simulink model "real_motor_model"  (R2023b)
settings: Solver=FixedStepAuto  StartTime=0.0  StopTime=2  FixedStep=0.0005  RelTol=1e-3
values from neighbouring files (symbols this model uses):
  dm = 0.0068    [params.m]
  Jm = 0.0104    [params.m]
settings Model: Creator=matte  LastModifiedBy=86180
settings SolverCC: AlgebraicLoopSolver=TrustRegion
settings DebuggingCC: ArithmeticOperatorsInVariantConditions=warning
settings SFSimCC: LegacyBehaviorForPersistentVarInContinuousTime=on  CustomCodeUndefinedFunction=UseInterfaceOnly

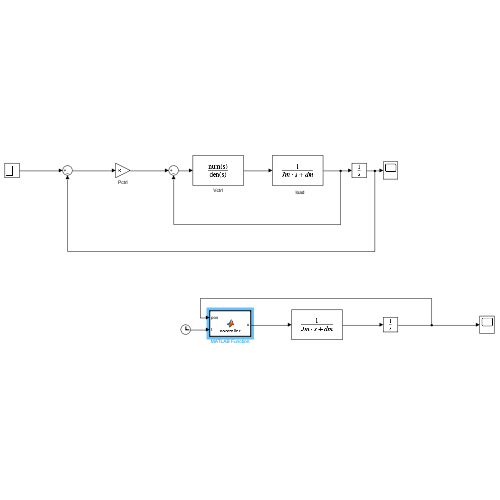
[thumbnail: Simulink's stored preview of the top-level diagram]
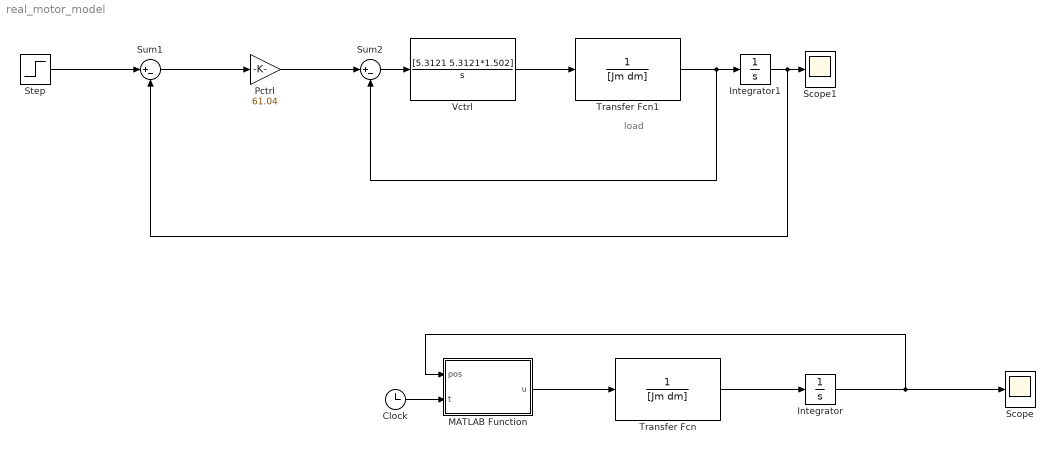
== system real_motor_model ==
  note: load
  Clock : Clock
  Integrator : Integrator
  Integrator1 : Integrator
  MATLAB Function : MATLAB Function  TreatAsAtomicUnit=on
  Pctrl : Gain  Gain=61.04
  Scope : Scope
  Scope1 : Scope
  Step : Step  SampleTime=0
  Sum1 : Sum  Inputs=|+-
  Sum2 : Sum  Inputs=|+-
  Transfer Fcn : TransferFcn  Denominator=[Jm dm]
  Transfer Fcn1 : TransferFcn  Denominator=[Jm dm]
  Vctrl : TransferFcn  Numerator=[5.3121 5.3121*1.502]  Denominator=[1 0]
  wires:
  Integrator/1 -> MATLAB Function/1(pos), Scope/1
  Transfer Fcn/1 -> Integrator/1
  Clock/1 -> MATLAB Function/2(t)
  MATLAB Function/1(u) -> Transfer Fcn/1
  Transfer Fcn1/1 -> Sum2/2, Integrator1/1
  Step/1 -> Sum1/1
  Vctrl/1 -> Transfer Fcn1/1
  Sum2/1 -> Vctrl/1
  Integrator1/1 -> Sum1/2, Scope1/1
  Pctrl/1 -> Sum2/1
  Sum1/1 -> Pctrl/1

== matlab function real_motor_model/MATLAB Function ==
  data: pos input; u output; t input
function u = controller(pos, t)

persistent last_t;
persistent last_pos;
persistent i_vel_e;

if isempty(last_pos)
    last_pos =pos;
end

% One time variable initialization --------
if isempty(last_t)
    last_t = 0;
end
% ----------------------------------------

if isempty(i_vel_e)
    i_vel_e = 0;
end

dt = t - last_t;

% Dirty fix to avoid division by zero --------
if dt == 0
    dt = 1e-4;
end

% --------------------------------------------
% implement your controller here
% -------------------------------------------- 
ref = 1;
% pos_controller= 66.955;
% real motor
pos_controller= 62.381; % 30hz of vel controller , 9.48hz of pos controller
% pos_controller= 61.04; % 81.3hz of vel controller , 9.66hz of pos controller
vel = (pos-last_pos)/dt;
ref_vel=(ref-pos)*pos_controller;

vel_e = ref_vel - vel;
  % 
  % 0.056382 (s+0.0003498)
  % ----------------------
  %           s

%  real motor
  %   1.9735 (s+0.8183)
  % -----------------          30hz
  %         s

  % 62.381   9.48hz

  % 5.3121 (s+1.502)
  % ----------------       81.3hz
  %        s
  % 61.04  9.66hz
% Pv=0.056382;
% Iv=0.056382*0.0003498;
% % real motor
Pv=1.9735;
Iv=1.9735*0.8183; % % 30hz of vel controller , 9.48hz of pos controller
% Pv=5.3121;
% Iv=5.3121*1.502; % % 81.3hz of vel controller , 9.66hz of pos controller
i_vel_e = i_vel_e + vel_e*dt;
vel_controller= Pv*vel_e + Iv*i_vel_e;

u =vel_controller;
last_t = t;
last_pos=pos;
